simulink model "pll_stability_9bus"  (R2025b)
settings: Solver=ode23t  StartTime=0.0  StopTime=0.6  FixedStep=Ts  RelTol=1e-3  EnableMultiTasking=on
InitFcn:
  | proj_root = fileparts(get_param(bdroot, 'FileName'));
  | run(fullfile(proj_root, 'params.m'))
StopFcn:
  | run(fullfile(fileparts(get_param(bdroot, 'FileName')), 'scripts', 'export_sim_data.m'))
values from neighbouring files (symbols this model uses):
  C1 = 4.247098756978487e-05    (= 4.24709875698e-05)    [GridTiedInverterOptimalIData.m]    (also in params.m)
  den_notch_d = [1.0, -1.9198159829792367, 0.9417686752314415]    [params.m]
  Ki = 7075.557375636462 /4    (= 1768.88934391)    [GridTiedInverterOptimalIData.m]    (also in params.m)
  ki_pll = ki_pll * 0.2    (= 21164)    [params.m]
  Kp = 29.481489065151926 /4    (= 7.37037226629)    [GridTiedInverterOptimalIData.m]    (also in params.m)
  kp_pll = kp_pll * 0.2    (= 92)    [params.m]
  L1 = 0.03042088602562317    (= 0.0304208860256)    [GridTiedInverterOptimalIData.m]    (also in params.m)
  L2 = 0.0002889984172434201    (= 0.000288998417243)    [GridTiedInverterOptimalIData.m]    (also in params.m)
  num_notch_d = [0.9723401207349347, -1.9198159829792367, 0.9694285544965067]    [params.m]
  qsi = 0.707    [GridTiedInverterOptimalIData.m]    (also in params.m)
  Rd1 = 0.5734201923227409    (= 0.573420192323)    [GridTiedInverterOptimalIData.m]    (also in params.m)
  Rd2 = 0.0054474918270660385    (= 0.00544749182707)    [GridTiedInverterOptimalIData.m]    (also in params.m)
  Rd3 = 3.1228169353331086    (= 3.12281693533)    [GridTiedInverterOptimalIData.m]    (also in params.m)
  Ts = 5e-6    (= 5e-06)    [GridTiedInverterOptimalIData.m]    (also in params.m)
  Tsc = 2e-4    (= 0.0002)    [GridTiedInverterOptimalIData.m]    (also in params.m)
  Vcc = 90909.09090909091*1.5    (= 136363.636364)    [GridTiedInverterOptimalIData.m]    (also in params.m)
  wres = 9068.99682117109    (= 9068.99682117)    [GridTiedInverterOptimalIData.m]    (also in params.m)
libraries: nesl_utility x80, ee_lib x71, fl_lib x28, eeGeneralControl x9, eeTransforms x4, eeSmAC1C x3, eeSmPSS1A x3, simulink x3, eeSinusoidalMeasurement x1
(part 2 of 3)

== system pll_stability_9bus/Gen2@Bus2 PV 1.025 pu 163 MW ==
  AVR and Exciter : Subsystem
  Bus Creator : BusCreator  Inputs=3
  Gen2 : ee_lib/Electromechanical/Synchronous/Synchronous Machine Round Rotor  port_option=ee.enum.threePhasePort.composite  SRated=192 MW  VRated=18 kV  FRated=60 Hz  nPolePairs=1  param_option=ee.enum.sm.parameterization.standard  fieldCircuitParameterization_option=ee.enum.sm.fieldparameterization.current  baseEfd=92.95 V  baseIfd=100 A  zero_sequence=ee.enum.park.zerosequence.include  axes_param=ee.enum.rotorangle.qaxis  Ladu=1.6801  Laqu=1.62  L0=0.0399  Ll=0.0399  Ra=0.01  Lfd=0.2162  Rfd=8.558e-4  L1d=0.4343  R1d=0.0325  L1q=0.2635  R1q=0.0326  L2q=0.4627  R2q=0.0131  Xl=0.1  Xd=1.7199  Xq=1.6598  X0=0.1  Xdd=0.23  Xqd=0.378  Xddd=0.1728  Xqdd=0.192  d_option=ee.enum.circuit.open  Td0d=6 s  Tdd=1.3260 s  Td0dd=0.05 s  Tddd=0.0230 s  q_option=ee.enum.circuit.open  Tq0d=0.535 s  Tqd=0.3693 s  Tq0dd=0.04 s  Tqdd=0.0269 s  saturation_option=ee.enum.saturation.exclude  saturation_ifd=[0.0, 0.48, 0.76, 1.38, 1.79]  saturation_Vag=[0.0, 0.8, 1.08, 1.31, 1.4]  initialization_option=ee.enum.sm.initialization.steadystate  source_type=ee.enum.sm.load_flow_source_type.PV  Vmag0=18*1.025 kV  Vang0=0 deg  Pt0=163 MW  Qt0=0 V*A  minimum_pu=0.95  phase_search_range=[-30, 30] deg  gmin=1e-6 S  connection_option=ee.enum.Connection.wye  num_q_dampers=2  rotor_offset=-pi / 2 rad  pu_psid_specify=on  pu_psid_priority=High  pu_psid=0  pu_psid_nominal_specify=off  pu_psid_nominal_value=1  pu_psid_nominal_unit=1  pu_psiq_specify=on  pu_psiq_priority=High  pu_psiq=0  pu_psiq_nominal_specify=off  pu_psiq_nominal_value=1  pu_psiq_nominal_unit=1  pu_psifd_specify=on  pu_psifd_priority=High  pu_psifd=0  pu_psifd_nominal_specify=off  pu_psifd_nominal_value=1  pu_psifd_nominal_unit=1  pu_psi1d_specify=on  pu_psi1d_priority=High  pu_psi1d=0  pu_psi1d_nominal_specify=off  pu_psi1d_nominal_value=1  pu_psi1d_nominal_unit=1  pu_psi1q_specify=on  pu_psi1q_priority=High  pu_psi1q=0  pu_psi1q_nominal_specify=off  pu_psi1q_nominal_value=1  pu_psi1q_nominal_unit=1  pu_psi2q_specify=on  pu_psi2q_priority=High  pu_psi2q=0  pu_psi2q_nominal_specify=off  pu_psi2q_nominal_value=1  pu_psi2q_nominal_unit=1  angular_position_diff_specify=off  angular_position_diff_priority=None  angular_position_diff=0 deg  angular_position_diff_nominal_specify=off  angular_position_diff_nominal_value=1  angular_position_diff_nominal_unit=deg  Tmeas=298.15 K  alpha=3.93e-3 1/K  stator_thermal_mass=100 J/K  rotor_thermal_mass=200 J/K  temperatureA_specify=off  temperatureA_priority=High  temperatureA=25 degC  temperatureA_nominal_specify=off  temperatureA_nominal_value=1  temperatureA_nominal_unit=degC  temperatureB_specify=off  temperatureB_priority=High  temperatureB=25 degC  temperatureB_nominal_specify=off  temperatureB_nominal_value=1  temperatureB_nominal_unit=degC  temperatureC_specify=off  temperatureC_priority=High  temperatureC=25 degC  temperatureC_nominal_specify=off  temperatureC_nominal_value=1  temperatureC_nominal_unit=degC  temperatureR_specify=off  temperatureR_priority=High  temperatureR=25 degC  temperatureR_nominal_specify=off  temperatureR_nominal_value=1  temperatureR_nominal_unit=degC
      settings: InternalSimscapePortConfiguration="{\"Bottom\":[],\"Left\":[{\"id\":\"fd_p\",\"label\":\"fd+\",\"type\":\"foundation.electrical.electrical\"},{\"id\":\"fd_n\",\"label\":\"fd-\",\"type\":\"foundation.electrical.electrical\"},{\"id\":\"R\",\"label\":\"R\",\"type\":\"foundation.mechanical.rotational.rotational\"},{\"id\":\"C\",\"label\":\"C\",\"type\":\"foundation.mechanical.rotational.rotational\"}],\"Right\":[{\"id\":\"pu_output\",\"label\":\"pu\",\"type\":\"output\"},{\"id\":\"N\",\"label\":\"~\",\"type\":\"foundation.electrical.three_phase\"},{\"id\":\"n\",\"label\":\"n\",\"type\":\"foundation.electrical.electrical\"}],\"Top\":[]}"
  Gnd : fl_lib/Electrical/Electrical Elements/Electrical Reference
  Governor and Prime Mover : Subsystem
  PS-Simulink Converter1 : nesl_utility/PS-Simulink Converter  PhysicalDomain=network_engine_domain  SubClassName=ps_output  LeftPortType=input  RightPortType=output  PseudoPeriodic=off  Frequencies=[]  VectorFormat=1-D array  Unit=1  AffineConversion=off
  PS-Simulink Converter11 : nesl_utility/PS-Simulink Converter  PhysicalDomain=network_engine_domain  SubClassName=ps_output  LeftPortType=input  RightPortType=output  PseudoPeriodic=off  Frequencies=[]  VectorFormat=1-D array  Unit=1  AffineConversion=off
  PS-Simulink Converter12 : nesl_utility/PS-Simulink Converter  PhysicalDomain=network_engine_domain  SubClassName=ps_output  LeftPortType=input  RightPortType=output  PseudoPeriodic=off  Frequencies=[]  VectorFormat=1-D array  Unit=1  AffineConversion=off
  Rotor electrical angle : ee_lib/Electromechanical/Synchronous/Synchronous Machine Measurement  output_idx=19
      settings: InternalSimscapePortConfiguration="{\"Bottom\":[],\"Left\":[{\"id\":\"pu_input\",\"label\":\"pu\",\"type\":\"input\"}],\"Right\":[{\"id\":\"pu_output\",\"label\":\"o\",\"type\":\"output\"}],\"Top\":[]}"
  Rotor velocity : ee_lib/Electromechanical/Synchronous/Synchronous Machine Measurement  output_idx=4
      settings: InternalSimscapePortConfiguration="{\"Bottom\":[],\"Left\":[{\"id\":\"pu_input\",\"label\":\"pu\",\"type\":\"input\"}],\"Right\":[{\"id\":\"pu_output\",\"label\":\"o\",\"type\":\"output\"}],\"Top\":[]}"
  Terminal voltage : ee_lib/Electromechanical/Synchronous/Synchronous Machine Measurement  output_idx=14
      settings: InternalSimscapePortConfiguration="{\"Bottom\":[],\"Left\":[{\"id\":\"pu_input\",\"label\":\"pu\",\"type\":\"input\"}],\"Right\":[{\"id\":\"pu_output\",\"label\":\"o\",\"type\":\"output\"}],\"Top\":[]}"
  ConnGen : PMIOPort  Side=Right
  mGen : Outport
  wires:
  PS-Simulink Converter11/1 -> Bus Creator/1  "w"
  Bus Creator/1 -> mGen/1
  PS-Simulink Converter12/1 -> Bus Creator/2  "Vt"
  PS-Simulink Converter1/1 -> Bus Creator/3  "theta"
  connections:
  AVR and Exciter/RConn1 -- Gen2/LConn1
  AVR and Exciter/RConn2 -- Gen2/LConn2
  Gen2/LConn3 -- Governor and Prime Mover/RConn1
  Gen2/LConn4 -- Governor and Prime Mover/RConn2
  Gen2/RConn2 -- ConnGen/RConn1
  Gen2/RConn3 -- Gnd/LConn1
  Gen2/RConn1 -- AVR and Exciter/LConn1 -- Governor and Prime Mover/LConn1 -- Rotor electrical angle/LConn1 -- Rotor velocity/LConn1 -- Terminal voltage/LConn1
  PS-Simulink Converter11/LConn1 -- Rotor velocity/RConn1
  PS-Simulink Converter12/LConn1 -- Terminal voltage/RConn1
  Rotor electrical angle/RConn1 -- PS-Simulink Converter1/LConn1

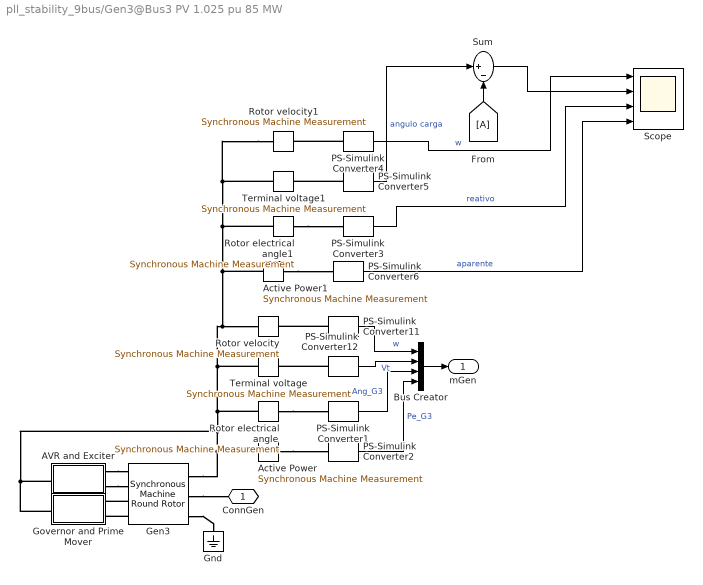
== system pll_stability_9bus/Gen3@Bus3 PV 1.025 pu 85 MW ==
  AVR and Exciter : Subsystem
  Active Power : ee_lib/Electromechanical/Synchronous/Synchronous Machine Measurement  output_idx=12
      settings: InternalSimscapePortConfiguration="{\"Bottom\":[],\"Left\":[{\"id\":\"pu_input\",\"label\":\"pu\",\"type\":\"input\"}],\"Right\":[{\"id\":\"pu_output\",\"label\":\"o\",\"type\":\"output\"}],\"Top\":[]}"
  Active Power1 : ee_lib/Electromechanical/Synchronous/Synchronous Machine Measurement  output_idx=11
      settings: InternalSimscapePortConfiguration="{\"Bottom\":[],\"Left\":[{\"id\":\"pu_input\",\"label\":\"pu\",\"type\":\"input\"}],\"Right\":[{\"id\":\"pu_output\",\"label\":\"o\",\"type\":\"output\"}],\"Top\":[]}"
  Bus Creator : BusCreator  Inputs=4
  From : From
  Gen3 : ee_lib/Electromechanical/Synchronous/Synchronous Machine Round Rotor  port_option=ee.enum.threePhasePort.composite  SRated=128 MW  VRated=13.8 kV  FRated=60 Hz  nPolePairs=1  param_option=ee.enum.sm.parameterization.standard  fieldCircuitParameterization_option=ee.enum.sm.fieldparameterization.current  baseEfd=92.95 V  baseIfd=100 A  zero_sequence=ee.enum.park.zerosequence.include  axes_param=ee.enum.rotorangle.qaxis  Ladu=1.5958  Laqu=1.5257  L0=0.0842  Ll=0.0842  Ra=0.01  Lfd=0.1715  Rfd=8.4749e-4  L1d=0.061  R1d=0.0108  L1q=0.1726  R1q=0.0222  L2q=0.3535  R2q=0.0144  Xl=0.095  Xd=1.68  Xq=1.61  X0=0.095  Xdd=0.2321  Xqd=0.32  Xddd=0.128  Xqdd=0.192  d_option=ee.enum.circuit.open  Td0d=5.89 s  Tdd=1.3260 s  Td0dd=0.05 s  Tddd=0.0230 s  q_option=ee.enum.circuit.open  Tq0d=0.6 s  Tqd=0.3693 s  Tq0dd=0.04 s  Tqdd=0.0269 s  saturation_option=ee.enum.saturation.exclude  saturation_ifd=[0.0, 0.48, 0.76, 1.38, 1.79]  saturation_Vag=[0.0, 0.8, 1.08, 1.31, 1.4]  initialization_option=ee.enum.sm.initialization.steadystate  source_type=ee.enum.sm.load_flow_source_type.PV  Vmag0=13.8*1.025 kV  Vang0=0 deg  Pt0=85 MW  Qt0=0 V*A  minimum_pu=0.95  phase_search_range=[-30, 30] deg  gmin=1e-6 S  connection_option=ee.enum.Connection.wye  num_q_dampers=2  rotor_offset=-pi / 2 rad  pu_psid_specify=on  pu_psid_priority=High  pu_psid=0  pu_psid_nominal_specify=off  pu_psid_nominal_value=1  pu_psid_nominal_unit=1  pu_psiq_specify=on  pu_psiq_priority=High  pu_psiq=0  pu_psiq_nominal_specify=off  pu_psiq_nominal_value=1  pu_psiq_nominal_unit=1  pu_psifd_specify=on  pu_psifd_priority=High  pu_psifd=0  pu_psifd_nominal_specify=off  pu_psifd_nominal_value=1  pu_psifd_nominal_unit=1  pu_psi1d_specify=on  pu_psi1d_priority=High  pu_psi1d=0  pu_psi1d_nominal_specify=off  pu_psi1d_nominal_value=1  pu_psi1d_nominal_unit=1  pu_psi1q_specify=on  pu_psi1q_priority=High  pu_psi1q=0  pu_psi1q_nominal_specify=off  pu_psi1q_nominal_value=1  pu_psi1q_nominal_unit=1  pu_psi2q_specify=on  pu_psi2q_priority=High  pu_psi2q=0  pu_psi2q_nominal_specify=off  pu_psi2q_nominal_value=1  pu_psi2q_nominal_unit=1  angular_position_diff_specify=off  angular_position_diff_priority=High  angular_position_diff=0 deg  angular_position_diff_nominal_specify=off  angular_position_diff_nominal_value=1  angular_position_diff_nominal_unit=deg  Tmeas=298.15 K  alpha=3.93e-3 1/K  stator_thermal_mass=100 J/K  rotor_thermal_mass=200 J/K  temperatureA_specify=off  temperatureA_priority=High  temperatureA=25 degC  temperatureA_nominal_specify=off  temperatureA_nominal_value=1  temperatureA_nominal_unit=degC  temperatureB_specify=off  temperatureB_priority=High  temperatureB=25 degC  temperatureB_nominal_specify=off  temperatureB_nominal_value=1  temperatureB_nominal_unit=degC  temperatureC_specify=off  temperatureC_priority=High  temperatureC=25 degC  temperatureC_nominal_specify=off  temperatureC_nominal_value=1  temperatureC_nominal_unit=degC  temperatureR_specify=off  temperatureR_priority=High  temperatureR=25 degC  temperatureR_nominal_specify=off  temperatureR_nominal_value=1  temperatureR_nominal_unit=degC
      settings: InternalSimscapePortConfiguration="{\"Bottom\":[],\"Left\":[{\"id\":\"fd_p\",\"label\":\"fd+\",\"type\":\"foundation.electrical.electrical\"},{\"id\":\"fd_n\",\"label\":\"fd-\",\"type\":\"foundation.electrical.electrical\"},{\"id\":\"R\",\"label\":\"R\",\"type\":\"foundation.mechanical.rotational.rotational\"},{\"id\":\"C\",\"label\":\"C\",\"type\":\"foundation.mechanical.rotational.rotational\"}],\"Right\":[{\"id\":\"pu_output\",\"label\":\"pu\",\"type\":\"output\"},{\"id\":\"N\",\"label\":\"~\",\"type\":\"foundation.electrical.three_phase\"},{\"id\":\"n\",\"label\":\"n\",\"type\":\"foundation.electrical.electrical\"}],\"Top\":[]}"
  Gnd : fl_lib/Electrical/Electrical Elements/Electrical Reference
  Governor and Prime Mover : Subsystem
  PS-Simulink Converter{1..6,11..12} (8 alike) : nesl_utility/PS-Simulink Converter  PhysicalDomain=network_engine_domain  SubClassName=ps_output  LeftPortType=input  RightPortType=output  PseudoPeriodic=off  Frequencies=[]  VectorFormat=1-D array  Unit=1  AffineConversion=off
  Rotor electrical angle : ee_lib/Electromechanical/Synchronous/Synchronous Machine Measurement  output_idx=19
      settings: InternalSimscapePortConfiguration="{\"Bottom\":[],\"Left\":[{\"id\":\"pu_input\",\"label\":\"pu\",\"type\":\"input\"}],\"Right\":[{\"id\":\"pu_output\",\"label\":\"o\",\"type\":\"output\"}],\"Top\":[]}"
  Rotor electrical angle1 : ee_lib/Electromechanical/Synchronous/Synchronous Machine Measurement  output_idx=13
      settings: InternalSimscapePortConfiguration="{\"Bottom\":[],\"Left\":[{\"id\":\"pu_input\",\"label\":\"pu\",\"type\":\"input\"}],\"Right\":[{\"id\":\"pu_output\",\"label\":\"o\",\"type\":\"output\"}],\"Top\":[]}"
  Rotor velocity : ee_lib/Electromechanical/Synchronous/Synchronous Machine Measurement  output_idx=4
      settings: InternalSimscapePortConfiguration="{\"Bottom\":[],\"Left\":[{\"id\":\"pu_input\",\"label\":\"pu\",\"type\":\"input\"}],\"Right\":[{\"id\":\"pu_output\",\"label\":\"o\",\"type\":\"output\"}],\"Top\":[]}"
  Rotor velocity1 : ee_lib/Electromechanical/Synchronous/Synchronous Machine Measurement  output_idx=4
      settings: InternalSimscapePortConfiguration="{\"Bottom\":[],\"Left\":[{\"id\":\"pu_input\",\"label\":\"pu\",\"type\":\"input\"}],\"Right\":[{\"id\":\"pu_output\",\"label\":\"o\",\"type\":\"output\"}],\"Top\":[]}"
  Scope : Scope  NumInputPorts=4
      settings: ActiveDisplayYMinimum=0.992134056706686  ActiveDisplayYMaximum=1.0008746376390321  DataLoggingVariableName=ScopeData28
  Sum : Sum  Inputs=|+-
  Terminal voltage : ee_lib/Electromechanical/Synchronous/Synchronous Machine Measurement  output_idx=14
      settings: InternalSimscapePortConfiguration="{\"Bottom\":[],\"Left\":[{\"id\":\"pu_input\",\"label\":\"pu\",\"type\":\"input\"}],\"Right\":[{\"id\":\"pu_output\",\"label\":\"o\",\"type\":\"output\"}],\"Top\":[]}"
  Terminal voltage1 : ee_lib/Electromechanical/Synchronous/Synchronous Machine Measurement  output_idx=18
      settings: InternalSimscapePortConfiguration="{\"Bottom\":[],\"Left\":[{\"id\":\"pu_input\",\"label\":\"pu\",\"type\":\"input\"}],\"Right\":[{\"id\":\"pu_output\",\"label\":\"o\",\"type\":\"output\"}],\"Top\":[]}"
  ConnGen : PMIOPort  Side=Right
  mGen : Outport
  wires:
  PS-Simulink Converter1/1 -> Bus Creator/3  "Ang_G3"
  PS-Simulink Converter12/1 -> Bus Creator/2  "Vt"
  Bus Creator/1 -> mGen/1
  PS-Simulink Converter11/1 -> Bus Creator/1  "w"
  PS-Simulink Converter2/1 -> Bus Creator/4  "Pe_G3"
  PS-Simulink Converter5/1 -> Sum/1  "angulo carga"
  PS-Simulink Converter4/1 -> Scope/1  "w"
  PS-Simulink Converter3/1 -> Scope/3  "reativo"
  PS-Simulink Converter6/1 -> Scope/4  "aparente"
  From/1 -> Sum/2
  Sum/1 -> Scope/2
  connections:
  Rotor electrical angle/RConn1 -- PS-Simulink Converter1/LConn1
  PS-Simulink Converter12/LConn1 -- Terminal voltage/RConn1
  PS-Simulink Converter11/LConn1 -- Rotor velocity/RConn1
  Rotor velocity1/LConn1 -- Terminal voltage1/LConn1 -- Rotor electrical angle1/LConn1 -- Rotor velocity/LConn1 -- Terminal voltage/LConn1 -- Gen3/RConn1 -- Active Power/LConn1 -- AVR and Exciter/LConn1 -- Governor and Prime Mover/LConn1 -- Rotor electrical angle/LConn1 -- Active Power1/LConn1
  Gen3/RConn3 -- Gnd/LConn1
  Gen3/RConn2 -- ConnGen/RConn1
  Gen3/LConn4 -- Governor and Prime Mover/RConn2
  Gen3/LConn3 -- Governor and Prime Mover/RConn1
  AVR and Exciter/RConn2 -- Gen3/LConn2
  AVR and Exciter/RConn1 -- Gen3/LConn1
  Active Power/RConn1 -- PS-Simulink Converter2/LConn1
  Active Power1/RConn1 -- PS-Simulink Converter6/LConn1
  PS-Simulink Converter4/LConn1 -- Rotor velocity1/RConn1
  PS-Simulink Converter5/LConn1 -- Terminal voltage1/RConn1
  Rotor electrical angle1/RConn1 -- PS-Simulink Converter3/LConn1

== system pll_stability_9bus/Scope ==
  BusElementIn : Inport  PortName=mGen1  Element=w
  BusElementIn1 : Inport  PortName=mGen1  Element=Vt
  BusElementIn3 : Inport  Port=2  PortName=mGen3  Element=Vt
  BusElementIn5 : Inport  Port=2  PortName=mGen3  Element=w
  Mux : Mux  Inputs=2
  Mux1 : Mux  Inputs=2
  Scope : Scope  NumInputPorts=2
      settings: ActiveDisplayYMinimum=0.30512027523637242  ActiveDisplayYMaximum=1.3392045145647005
  wires:
  BusElementIn/1 -> Mux/1
  BusElementIn1/1 -> Mux1/1
  BusElementIn3/1 -> Mux1/2
  Mux1/1 -> Scope/1  "Terminal voltages [p.u.]"
  Mux/1 -> Scope/2  "Rotor speeds [p.u.]"
  BusElementIn5/1 -> Mux/2

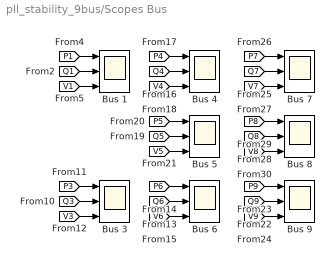
== system pll_stability_9bus/Scopes Bus ==
  Bus {1,3..9} (8 alike) : Scope  NumInputPorts=3
      Bus 1 settings: ActiveDisplayYMinimum=-49.114456824665893  ActiveDisplayYMaximum=442.03011142199318  DataLoggingVariableName=ScopeData11
      Bus 3 settings: ActiveDisplayYMinimum=-59.99075912656123  ActiveDisplayYMaximum=266.60428494941306  DataLoggingVariableName=ScopeData10
      Bus 4 settings: ActiveDisplayYMinimum=-38.55667965898116  ActiveDisplayYMaximum=347.01011693083052  DataLoggingVariableName=ScopeData14
      Bus 5 settings: ActiveDisplayYMinimum=-192.77982685772625  ActiveDisplayYMaximum=116.10526480167731  DataLoggingVariableName=ScopeData12
      Bus 6 settings: ActiveDisplayYMinimum=-45.726697361068808  ActiveDisplayYMaximum=76.089380993056864  DataLoggingVariableName=ScopeData13
      Bus 7 settings: ActiveDisplayYMinimum=-344.11330563303079  ActiveDisplayYMaximum=223.61219150109264  DataLoggingVariableName=ScopeData17
      Bus 8 settings: ActiveDisplayYMinimum=-150.38081880811259  ActiveDisplayYMaximum=115.04879751678179  DataLoggingVariableName=ScopeData15
      Bus 9 settings: ActiveDisplayYMinimum=-29.497454320573244  ActiveDisplayYMaximum=265.47708888515928  DataLoggingVariableName=ScopeData16
  wires:
  [V4] -> Bus 4/3
  [Q9] -> Bus 9/2
  [V6] -> Bus 6/3
  [V9] -> Bus 9/3
  [P5] -> Bus 5/1
  [Q1] -> Bus 1/2
  [Q8] -> Bus 8/2
  [P6] -> Bus 6/1
  [P4] -> Bus 4/1
  [V5] -> Bus 5/3
  [P9] -> Bus 9/1
  [V1] -> Bus 1/3
  [Q5] -> Bus 5/2
  [P7] -> Bus 7/1
  [Q6] -> Bus 6/2
  [Q4] -> Bus 4/2
  [P8] -> Bus 8/1
  [P1] -> Bus 1/1
  [V8] -> Bus 8/3
  [V7] -> Bus 7/3
  [Q7] -> Bus 7/2
  [Q3] -> Bus 3/2
  [P3] -> Bus 3/1
  [V3] -> Bus 3/3

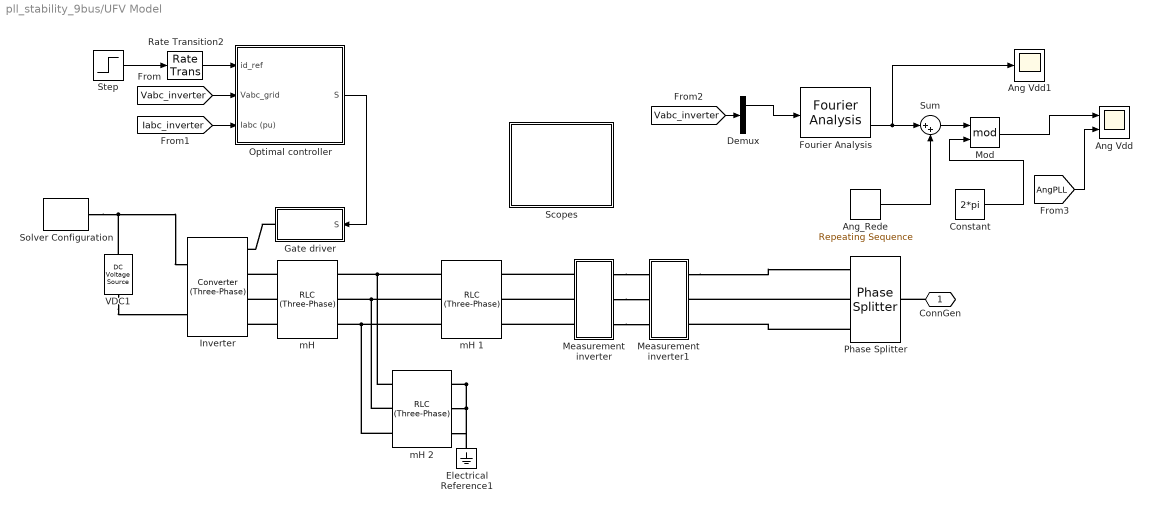
== system pll_stability_9bus/UFV Model ==
  " mH " : ee_lib/Passive/RLC Assemblies/RLC (Three-Phase)  port_option=ee.enum.threePhasePort.expanded  component_structure=ee.enum.rlc.structure.SeriesRL  R=Rd1 Ohm  L=L1 H  C=1 F  R_parasitic=1e-6 Ohm  G_parasitic=1e-6 1/Ohm  IL_specify=on  IL_priority=High  IL=[0, 0, 0] A  IL_nominal_specify=off  IL_nominal_value=1  IL_nominal_unit=A  VC_specify=on  VC_priority=High  VC=[0, 0, 0] V  VC_nominal_specify=off  VC_nominal_value=1  VC_nominal_unit=V
      settings: InternalSimscapePortConfiguration="{\"Bottom\":[],\"Left\":[{\"id\":\"a1\",\"label\":\"a1\",\"type\":\"foundation.electrical.electrical\"},{\"id\":\"b1\",\"label\":\"b1\",\"type\":\"foundation.electrical.electrical\"},{\"id\":\"c1\",\"label\":\"c1\",\"type\":\"foundation.electrical.electrical\"}],\"Right\":[{\"id\":\"a2\",\"label\":\"a2\",\"type\":\"foundation.electrical.electrical\"},{\"id\":\"b2\",\"label\":\"b2\",\"type\":\"foundation.electrical.electrical\"},{\"id\":\"c2\",\"label\":\"c2\",\"type\":\"foundation.electrical.electrical\"}],\"Top\":[]}"
  " mH 1" : ee_lib/Passive/RLC Assemblies/RLC (Three-Phase)  port_option=ee.enum.threePhasePort.expanded  component_structure=ee.enum.rlc.structure.SeriesRL  R=Rd2 Ohm  L=L2 H  C=1 F  R_parasitic=1e-6 Ohm  G_parasitic=1e-6 1/Ohm  IL_specify=on  IL_priority=High  IL=[0, 0, 0] A  IL_nominal_specify=off  IL_nominal_value=1  IL_nominal_unit=A  VC_specify=on  VC_priority=High  VC=[0, 0, 0] V  VC_nominal_specify=off  VC_nominal_value=1  VC_nominal_unit=V
      settings: InternalSimscapePortConfiguration="{\"Bottom\":[],\"Left\":[{\"id\":\"a1\",\"label\":\"a1\",\"type\":\"foundation.electrical.electrical\"},{\"id\":\"b1\",\"label\":\"b1\",\"type\":\"foundation.electrical.electrical\"},{\"id\":\"c1\",\"label\":\"c1\",\"type\":\"foundation.electrical.electrical\"}],\"Right\":[{\"id\":\"a2\",\"label\":\"a2\",\"type\":\"foundation.electrical.electrical\"},{\"id\":\"b2\",\"label\":\"b2\",\"type\":\"foundation.electrical.electrical\"},{\"id\":\"c2\",\"label\":\"c2\",\"type\":\"foundation.electrical.electrical\"}],\"Top\":[]}"
  " mH 2" : ee_lib/Passive/RLC Assemblies/RLC (Three-Phase)  port_option=ee.enum.threePhasePort.expanded  component_structure=ee.enum.rlc.structure.ParallelRC  R=Rd3 Ohm  L=0.002 H  C=C1 F  R_parasitic=1e-6 Ohm  G_parasitic=1e-6 1/Ohm  IL_specify=on  IL_priority=High  IL=[0, 0, 0] A  IL_nominal_specify=off  IL_nominal_value=1  IL_nominal_unit=A  VC_specify=on  VC_priority=High  VC=[0, 0, 0] V  VC_nominal_specify=off  VC_nominal_value=1  VC_nominal_unit=V
      settings: InternalSimscapePortConfiguration="{\"Bottom\":[],\"Left\":[{\"id\":\"a1\",\"label\":\"a1\",\"type\":\"foundation.electrical.electrical\"},{\"id\":\"b1\",\"label\":\"b1\",\"type\":\"foundation.electrical.electrical\"},{\"id\":\"c1\",\"label\":\"c1\",\"type\":\"foundation.electrical.electrical\"}],\"Right\":[{\"id\":\"a2\",\"label\":\"a2\",\"type\":\"foundation.electrical.electrical\"},{\"id\":\"b2\",\"label\":\"b2\",\"type\":\"foundation.electrical.electrical\"},{\"id\":\"c2\",\"label\":\"c2\",\"type\":\"foundation.electrical.electrical\"}],\"Top\":[]}"
  Ang Vdd : Scope  NumInputPorts=2
      settings: ActiveDisplayYMinimum=-0.78537822507117583  ActiveDisplayYMaximum=7.068404025640584  DataLoggingVariableName=ScopeData8
  Ang Vdd1 : Scope
      settings: ActiveDisplayYMinimum=-3.9268785604995653  ActiveDisplayYMaximum=3.9266971999008624  DataLoggingVariableName=ScopeData25
  Ang_Rede : simulink/Sources/Repeating Sequence  rep_seq_t=[0 1/60]  rep_seq_y=[0 2*pi]
  Constant : Constant  Value=2*pi
  Demux : Demux  Outputs=3
  Electrical Reference1 : fl_lib/Electrical/Electrical Elements/Electrical Reference
  Fourier Analysis : eeGeneralControl/Fourier Analysis  f=60  n=[1]  M0=1  Ph0=0  BufferSize=8192  Ts=-1
      settings: LibrarySourceBlock=ee_sl_lib/General Control/Fourier Analysis
  Gate driver : Subsystem
  Inverter : ee_lib/Semiconductors & Converters/Converters/Converter (Three-Phase)  port_option=ee.enum.threePhasePort.expanded  fidelity_option=ee.enum.converters.fidelity.detailed  device_type=ee.enum.converters.switchingdevice.ideal  showThermalPort=false  K=0  Vth=0.5 V  Vgt=1e-3 V  Vgt_off=-1 V  Ih=1 A  Vf=0.8 V  Ron=1e-3 Ohm  Rds=0.001 Ohm  Goff=2e-4 1/Ohm  Eon_scalar=22.86e-3 J  Eoff_scalar=17.14e-3 J  Eoff_natural_commutation=10e-3 J  Voff=300 V  Iout_scalar=600 A  onCurrentMeasDelay=0 s  useCurrentFromPreviousCycle=false  useVoltageFromPreviousCycle=false  diode_param=ee.enum.converters.protectiondiode.nodynamics  diode_Vf=0.8 V  diode_Ron=0.001 Ohm  diode_Goff=1e-5 1/Ohm  diode_C=50 nF  diode_iRM=-235 A  diode_iF=300 A  diode_idot=-50 A/us  diode_trr_param=ee.enum.converters.diodetrr.trr_factor  diode_trr_factor=3  diode_trr=15 us  diode_Qrr=1.5e+3 s*uA  diode_rec_loss_model=ee.enum.diode.reverseRecoveryModel.fixed  diode_ErecVal=0 J  diode_scaleWithIandV=false  diode_ErecMat=zeros(2, 3) J  diode_TjrecVec=[298.15, 398.15] K  diode_IfrecVec=[.1, 1, 10] A  diode_IrecVal=10 A  diode_VrecVal=10 V  diode_tFilter=1 / 1000 / 100 s  thermal_network_parameterization=ee.enum.thermalNetworkTopology.external  Rth=[.08, .5] K/W  Rth_Cauer=[.08, .1, .5] K/W  Rth_Foster=[.08, .14, .22, .16] K/W  thermal_mass_parameterization=ee.enum.thermalNetwork.timeconstant  thermal_mass=[.01, .5] J/K  thermal_mass_Cauer=[.01, .1, .5] J/K  thermal_mass_Foster=[.001, .005, .05, .5] J/K  thermal_time_constant=[.001, .2] s  thermal_time_constant_Cauer=[.001, .1, .2] s  thermal_time_constant_Foster=[7e-05, .0007, .01, .08] s  thermal_mass_initial_temperatures=[25, 25] degC  thermal_mass_initial_temperatures_Cauer=[25, 25, 25] degC  junction_thermal_mass=0.01 J/K  Tvec_initial_Foster=[25, 25, 25, 25] degC  snubber_type=ee.enum.converters.snubber.exclude  Cs=1e-7 F  Rs=0.1 Ohm  Vce_loss=[0, 150, 300] V
      settings: InternalSimscapePortConfiguration="{\"Bottom\":[],\"Left\":[{\"id\":\"G\",\"label\":\"G\",\"type\":\"foundation.electrical.twelve_phase\"},{\"id\":\"a\",\"label\":\"a\",\"type\":\"foundation.electrical.electrical\"},{\"id\":\"b\",\"label\":\"b\",\"type\":\"foundation.electrical.electrical\"},{\"id\":\"c\",\"label\":\"c\",\"type\":\"foundation.electrical.electrical\"}],\"Right\":[{\"id\":\"p\",\"label\":\"+\",\"type\":\"foundation.electrical.electrical\"},{\"id\":\"n\",\"label\":\"-\",\"type\":\"foundation.electrical.electrical\"}],\"Top\":[]}"
  Measurement inverter : Subsystem
  Measurement inverter1 : Subsystem
  Mod : Math  Operator=mod
  Optimal controller : Subsystem
  Phase Splitter : ee_lib/Connectors & References/Phase Splitter
  Rate Transition2 : RateTransition  OutPortSampleTime=Tsc
  Scopes : Subsystem
  Solver Configuration : nesl_utility/Solver Configuration  PhysicalDomain=network_engine_domain  SubClassName=solver  LeftPortType=input  RightPortType=generic  Tones=[]  Harmonics=[]  SimulateNoise=off  Profile=off  UseLocalSampling=off  EnableSwitchedLinearOptims=on  FrequencyDomain=off  UseCCode=off  RelTol=0.001  AbsTol=1e-06  MinStep=1e-09  ToWorkspace=off  RevertToSquareIcSolve=off  NumHomotopyIterations=100  PhasorMode=off  PhasorModeNumHarmonics=1  ConsistencySolver=NEWTON_FTOL  IndexReductionMethod=DerivativeReplacement  DoDC=off  ResidualTolerance=1e-09  ConsistencyTolSource=GLOBAL  ConsistencyAbsTol=0.001  ConsistencyRelTol=0.001  ConsistencyTolFactor=0.001  UseLocalSolver=on  LocalSolverChoice=NE_BACKWARD_EULER_ADVANCER  ResolveIndetEquations=on  FunctionEvalNumThread=1  LocalSolverSampleTime=Ts  DoFixedCost=off  MaxNonlinIter=3  MaxModeIter=2  ComputeImpulses=off  ImpulseIterations=1  LinearAlgebra=auto  LinearAlgebraNumThread=0  EquationFormulation=NE_TIME_EF  DelaysMemoryBudget=1024  AutomaticFiltering=on  FilteringTimeConstant=0.001  PartitionStorageMethod=AS_NEEDED  PartitionMemoryBudget=1024  PartitionMethod=FAST  MultibodyUseLocalSolver=off  MultibodyLocalSolverChoice=ODE1  MultibodyLocalSolverSampleTime=0.001
  Step : Step  Time=0.01  SampleTime=0
  Sum : Sum  Inputs=|++
  VDC1 : fl_lib/Electrical/Electrical Sources/DC Voltage Source  v0=Vcc*1.7 V
  ConnGen : PMIOPort  Side=Right
  wires:
  [Iabc_inverter] -> Optimal controller/3(Iabc (pu))
  [Vabc_inverter] -> Optimal controller/2(Vabc_grid)
  Rate Transition2/1 -> Optimal controller/1(id_ref)
  Step/1 -> Rate Transition2/1
  Optimal controller/1(S) -> Gate driver/1(S)
  [Vabc_inverter] -> Demux/1
  Demux/1 -> Fourier Analysis/1
  Fourier Analysis/2 -> Ang Vdd1/1, Sum/1
  Ang_Rede/1 -> Sum/2
  Sum/1 -> Mod/1
  Mod/1 -> Ang Vdd/1
  Constant/1 -> Mod/2
  [AngPLL] -> Ang Vdd/2
  connections:
  " mH 2"/LConn3 -- " mH "/RConn3 -- " mH 1"/LConn3
  " mH 2"/RConn1 -- " mH 2"/RConn2 -- Electrical Reference1/LConn1 -- " mH 2"/RConn3
  " mH 2"/LConn2 -- " mH "/RConn2 -- " mH 1"/LConn2
  Measurement inverter/LConn3 -- " mH 1"/RConn3
  " mH "/LConn2 -- Inverter/LConn3
  Solver Configuration/RConn1 -- Inverter/RConn1 -- VDC1/LConn1
  " mH 2"/LConn1 -- " mH "/RConn1 -- " mH 1"/LConn1
  Measurement inverter/RConn1 -- Measurement inverter1/LConn1
  Measurement inverter/RConn3 -- Measurement inverter1/LConn3
  " mH "/LConn1 -- Inverter/LConn2
  Measurement inverter/LConn1 -- " mH 1"/RConn1
  Gate driver/RConn1 -- Inverter/LConn1
  Phase Splitter/RConn3 -- Measurement inverter1/RConn3
  VDC1/RConn1 -- Inverter/RConn2
  " mH "/LConn3 -- Inverter/LConn4
  Measurement inverter1/RConn1 -- Phase Splitter/RConn1
  Phase Splitter/RConn2 -- Measurement inverter1/RConn2
  Measurement inverter/RConn2 -- Measurement inverter1/LConn2
  Measurement inverter/LConn2 -- " mH 1"/RConn2
  ConnGen/RConn1 -- Phase Splitter/LConn1

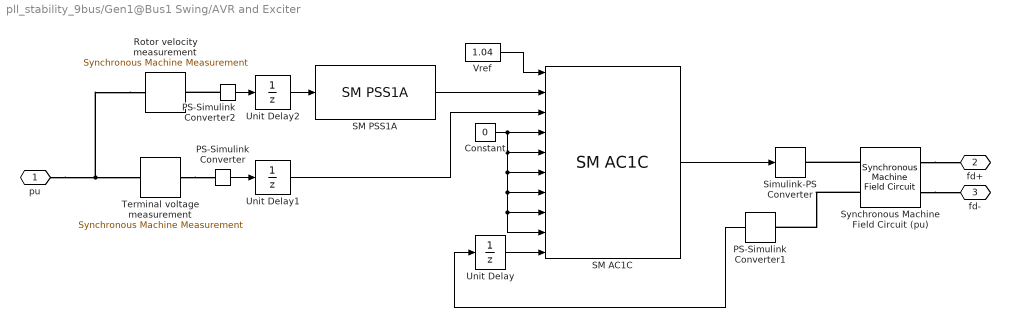
== system pll_stability_9bus/Gen1@Bus1 Swing/AVR and Exciter ==
  Constant : Constant  Value=0
  PS-Simulink Converter : nesl_utility/PS-Simulink Converter  PhysicalDomain=network_engine_domain  SubClassName=ps_output  LeftPortType=input  RightPortType=output  PseudoPeriodic=off  Frequencies=[]  VectorFormat=1-D array  Unit=1  AffineConversion=off
  PS-Simulink Converter1 : nesl_utility/PS-Simulink Converter  PhysicalDomain=network_engine_domain  SubClassName=ps_output  LeftPortType=input  RightPortType=output  PseudoPeriodic=off  Frequencies=[]  VectorFormat=1-D array  Unit=1  AffineConversion=off
  PS-Simulink Converter2 : nesl_utility/PS-Simulink Converter  PhysicalDomain=network_engine_domain  SubClassName=ps_output  LeftPortType=input  RightPortType=output  PseudoPeriodic=off  Frequencies=[]  VectorFormat=1-D array  Unit=1  AffineConversion=off
  Rotor velocity measurement : ee_lib/Electromechanical/Synchronous/Synchronous Machine Measurement  output_idx=4
      settings: InternalSimscapePortConfiguration="{\"Bottom\":[],\"Left\":[{\"id\":\"pu_input\",\"label\":\"pu\",\"type\":\"input\"}],\"Right\":[{\"id\":\"pu_output\",\"label\":\"o\",\"type\":\"output\"}],\"Top\":[]}"
  SM AC1C : eeSmAC1C/SM AC1C  E_FD0=1.08614  Ts=Ts  R_C=0  X_C=0  T_R=0  K_A=400  T_A=0.02  T_B=0  T_C=0  K_F=0.03  T_F=1  V_Amax=14.5  V_Amin=-14.5  E_FEmax=6.03  E_FEmin=-5.43  oelInputLocation=Unused  uelInputLocation=Unused  sclInputLocation=Unused  K_E=1  T_E=0.8  K_C=0.2  K_D=0.38  E_1=4.18  S_E_E1=0.1  E_2=3.14  S_E_E2=0.03  V_FEmax=99  V_Emin=0
  SM PSS1A : eeSmPSS1A/SM PSS1A  K_S=3.15  A_1=0  A_2=0  T_1=0  T_2=0  T_3=0.32  T_4=0.016  T_5=1  T_6=0.0106  V_STmax=0.09  V_STmin=-0.09  Ts=Ts
  Simulink-PS Converter : nesl_utility/Simulink-PS Converter  PhysicalDomain=network_engine_domain  SubClassName=ps_input  LeftPortType=input  RightPortType=output  PseudoPeriodic=off  Frequencies=[]  NoiseDistribution=none  NoiseParameters=[]  Unit=1  AffineConversion=off  FilteringAndDerivatives=provide  SimscapeFilterOrder=1  InputFilterTimeConstant=0.001  UdotUserProvided=0
  Synchronous Machine Field Circuit (pu) : ee_lib/Electromechanical/Synchronous/Synchronous Machine Field Circuit  unit_option=ee.enum.unit.pu  SRated=247.5 MW  FRated=60 Hz  fieldCircuitParameterization_option=ee.enum.sm.fieldparameterization.current  baseEfd=92.95 V  baseIfd=100 A  parameterization_option=ee.enum.sm.parameterization.standard  Ladu=0.2725  Rfd=1.0656e-4  Xl=0.0832  Xd=0.3614  Xdd=0.1505  Xddd=0.0990  d_option=ee.enum.circuit.open  Td0d=8.96 s  Tdd=1.3260 s  Td0dd=0.05 s  Tddd=0.0230 s
      settings: InternalSimscapePortConfiguration="{\"Bottom\":[],\"Left\":[{\"id\":\"Efd_pu\",\"label\":\"Efd_pu\",\"type\":\"input\"},{\"id\":\"Ifd_pu\",\"label\":\"Ifd_pu\",\"type\":\"output\"}],\"Right\":[{\"id\":\"fd_p\",\"label\":\"fd+\",\"type\":\"foundation.electrical.electrical\"},{\"id\":\"fd_n\",\"label\":\"fd-\",\"type\":\"foundation.electrical.electrical\"}],\"Top\":[]}"
  Terminal voltage measurement : ee_lib/Electromechanical/Synchronous/Synchronous Machine Measurement  output_idx=14
      settings: InternalSimscapePortConfiguration="{\"Bottom\":[],\"Left\":[{\"id\":\"pu_input\",\"label\":\"pu\",\"type\":\"input\"}],\"Right\":[{\"id\":\"pu_output\",\"label\":\"o\",\"type\":\"output\"}],\"Top\":[]}"
  Unit Delay : UnitDelay  InitialCondition=1.08614  SampleTime=Ts  HasFrameUpgradeWarning=on
  Unit Delay1 : UnitDelay  InitialCondition=1.04  SampleTime=Ts  HasFrameUpgradeWarning=on
  Unit Delay2 : UnitDelay  InitialCondition=1  SampleTime=Ts  HasFrameUpgradeWarning=on
  Vref : Constant  Value=1.04
  pu : PMIOPort  Side=Left
  fd+ : PMIOPort  Port=2  Side=Right
  fd- : PMIOPort  Port=3  Side=Right
  wires:
  Unit Delay2/1 -> SM PSS1A/1
  PS-Simulink Converter2/1 -> Unit Delay2/1
  Unit Delay1/1 -> SM AC1C/3
  Vref/1 -> SM AC1C/1
  Constant/1 -> SM AC1C/9, SM AC1C/8, SM AC1C/7, SM AC1C/6, SM AC1C/5, SM AC1C/4
  Unit Delay/1 -> SM AC1C/10
  SM AC1C/1 -> Simulink-PS Converter/1
  PS-Simulink Converter1/1 -> Unit Delay/1
  SM PSS1A/1 -> SM AC1C/2
  PS-Simulink Converter/1 -> Unit Delay1/1
  connections:
  PS-Simulink Converter2/LConn1 -- Rotor velocity measurement/RConn1
  Rotor velocity measurement/LConn1 -- Terminal voltage measurement/LConn1 -- pu/RConn1
  Terminal voltage measurement/RConn1 -- PS-Simulink Converter/LConn1
  Synchronous Machine Field Circuit (pu)/LConn1 -- Simulink-PS Converter/RConn1
  Synchronous Machine Field Circuit (pu)/LConn2 -- PS-Simulink Converter1/LConn1
  Synchronous Machine Field Circuit (pu)/RConn2 -- fd-/RConn1
  Synchronous Machine Field Circuit (pu)/RConn1 -- fd+/RConn1

== system pll_stability_9bus/Gen1@Bus1 Swing/Governor and Prime Mover ==
  "Governor and Prime Mover " : Subsystem  mask(Governor and Prime Mover){droop_percentage=5, Tg=0.15, Tch=0.3, pu_torque0=0.309487, Ts=Ts}
      mask prompts: droop_percentage "Percentage droop, (%)"; Tg "Time constant of governor, Tg (s)"; Tch "Time constant of main inlet volumes and steam chest, Tch (s)"; pu_torque0 "Initial torque, (pu)"; Ts "Sample time"
      mask help:
      | Implements a synchronous machine governor and prime mover. The prime mover is a non-reheat steam turbine.
      |
      | The input to the block is a per-unit synchronous machine measurement vector.
      |
      | R and C are mechanical rotational ports.
  Mechanical Power : ee_lib/Electromechanical/Mechanical/Machine Mechanical Power  power_sign=-1  SRated=247.5 MW  FRated=60 Hz  nPolePairs=20  inputUnit=ee.enum.unit.pu  torque_factor=2  inertia_option=2  J=27548 kg*m^2  H=6 W*s/(A*V)  damper_option=2  D=39.0509 N*m*s/rad  pu_D=0  initialization_option=2  fMechanical0=60 Hz  fElectrical0=60 Hz
      settings: InternalSimscapePortConfiguration="{\"Bottom\":[],\"Left\":[{\"id\":\"Pm_pu\",\"label\":\"pu\",\"type\":\"input\"}],\"Right\":[{\"id\":\"R\",\"label\":\"R\",\"type\":\"foundation.mechanical.rotational.rotational\"},{\"id\":\"C\",\"label\":\"C\",\"type\":\"foundation.mechanical.rotational.rotational\"}],\"Top\":[]}"
  PS-Simulink Converter : nesl_utility/PS-Simulink Converter  PhysicalDomain=network_engine_domain  SubClassName=ps_output  LeftPortType=input  RightPortType=output  PseudoPeriodic=off  Frequencies=[]  VectorFormat=1-D array  Unit=1  AffineConversion=off
  Pref : Constant  Value=76.4/247.5
  Rotor velocity measurement : ee_lib/Electromechanical/Synchronous/Synchronous Machine Measurement  output_idx=4
      settings: InternalSimscapePortConfiguration="{\"Bottom\":[],\"Left\":[{\"id\":\"pu_input\",\"label\":\"pu\",\"type\":\"input\"}],\"Right\":[{\"id\":\"pu_output\",\"label\":\"o\",\"type\":\"output\"}],\"Top\":[]}"
  Simulink-PS Converter : nesl_utility/Simulink-PS Converter  PhysicalDomain=network_engine_domain  SubClassName=ps_input  LeftPortType=input  RightPortType=output  PseudoPeriodic=off  Frequencies=[]  NoiseDistribution=none  NoiseParameters=[]  Unit=1  AffineConversion=off  FilteringAndDerivatives=provide  SimscapeFilterOrder=1  InputFilterTimeConstant=0.001  UdotUserProvided=0
  Unit Delay : UnitDelay  InitialCondition=1  SampleTime=Ts  HasFrameUpgradeWarning=on
  wref : Constant
  R : PMIOPort  Side=Right
  C : PMIOPort  Port=2  Side=Right
  pu : PMIOPort  Port=3  Side=Left
  wires:
  PS-Simulink Converter/1 -> Unit Delay/1
  Unit Delay/1 -> "Governor and Prime Mover "/3(w)
  Pref/1 -> "Governor and Prime Mover "/2(Pref)
  "Governor and Prime Mover "/1(Tm) -> Simulink-PS Converter/1
  wref/1 -> "Governor and Prime Mover "/1(wref)
  connections:
  PS-Simulink Converter/LConn1 -- Rotor velocity measurement/RConn1
  Mechanical Power/RConn1 -- R/RConn1
  pu/RConn1 -- Rotor velocity measurement/LConn1
  Mechanical Power/RConn2 -- C/RConn1
  Mechanical Power/LConn1 -- Simulink-PS Converter/RConn1

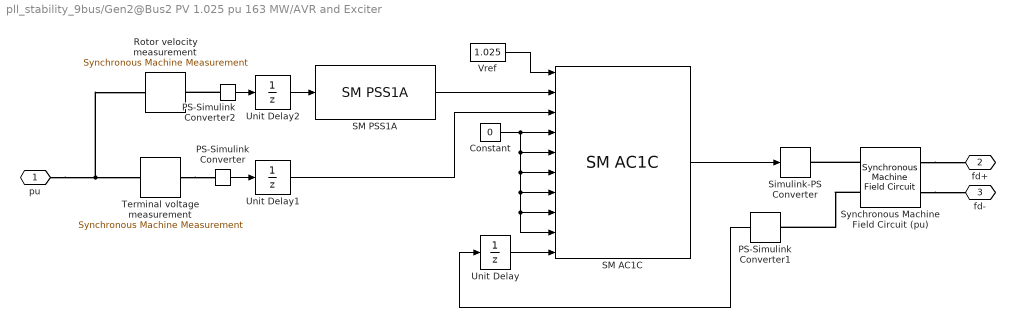
== system pll_stability_9bus/Gen2@Bus2 PV 1.025 pu 163 MW/AVR and Exciter ==
  Constant : Constant  Value=0
  PS-Simulink Converter : nesl_utility/PS-Simulink Converter  PhysicalDomain=network_engine_domain  SubClassName=ps_output  LeftPortType=input  RightPortType=output  PseudoPeriodic=off  Frequencies=[]  VectorFormat=1-D array  Unit=1  AffineConversion=off
  PS-Simulink Converter1 : nesl_utility/PS-Simulink Converter  PhysicalDomain=network_engine_domain  SubClassName=ps_output  LeftPortType=input  RightPortType=output  PseudoPeriodic=off  Frequencies=[]  VectorFormat=1-D array  Unit=1  AffineConversion=off
  PS-Simulink Converter2 : nesl_utility/PS-Simulink Converter  PhysicalDomain=network_engine_domain  SubClassName=ps_output  LeftPortType=input  RightPortType=output  PseudoPeriodic=off  Frequencies=[]  VectorFormat=1-D array  Unit=1  AffineConversion=off
  Rotor velocity measurement : ee_lib/Electromechanical/Synchronous/Synchronous Machine Measurement  output_idx=4
      settings: InternalSimscapePortConfiguration="{\"Bottom\":[],\"Left\":[{\"id\":\"pu_input\",\"label\":\"pu\",\"type\":\"input\"}],\"Right\":[{\"id\":\"pu_output\",\"label\":\"o\",\"type\":\"output\"}],\"Top\":[]}"
  SM AC1C : eeSmAC1C/SM AC1C  E_FD0=1.79759  Ts=Ts  R_C=0  X_C=0  T_R=0  K_A=400  T_A=0.02  T_B=0  T_C=0  K_F=0.03  T_F=1  V_Amax=14.5  V_Amin=-14.5  E_FEmax=6.03  E_FEmin=-5.43  oelInputLocation=Unused  uelInputLocation=Unused  sclInputLocation=Unused  K_E=1  T_E=0.8  K_C=0.2  K_D=0.38  E_1=4.18  S_E_E1=0.1  E_2=3.14  S_E_E2=0.03  V_FEmax=99  V_Emin=0
  SM PSS1A : eeSmPSS1A/SM PSS1A  K_S=3.15  A_1=0  A_2=0  T_1=0  T_2=0  T_3=0.32  T_4=0.016  T_5=1  T_6=0.0106  V_STmax=0.09  V_STmin=-0.09  Ts=Ts
  Simulink-PS Converter : nesl_utility/Simulink-PS Converter  PhysicalDomain=network_engine_domain  SubClassName=ps_input  LeftPortType=input  RightPortType=output  PseudoPeriodic=off  Frequencies=[]  NoiseDistribution=none  NoiseParameters=[]  Unit=1  AffineConversion=off  FilteringAndDerivatives=provide  SimscapeFilterOrder=1  InputFilterTimeConstant=0.001  UdotUserProvided=0
  Synchronous Machine Field Circuit (pu) : ee_lib/Electromechanical/Synchronous/Synchronous Machine Field Circuit  unit_option=ee.enum.unit.pu  SRated=192 MW  FRated=60 Hz  fieldCircuitParameterization_option=ee.enum.sm.fieldparameterization.current  baseEfd=92.95 V  baseIfd=100 A  parameterization_option=ee.enum.sm.parameterization.standard  Ladu=1.6801  Rfd=8.558e-4  Xl=0.1  Xd=1.7199  Xdd=0.23  Xddd=0.1728  d_option=ee.enum.circuit.open  Td0d=6 s  Tdd=1.3260 s  Td0dd=0.05 s  Tddd=0.0230 s
      settings: InternalSimscapePortConfiguration="{\"Bottom\":[],\"Left\":[{\"id\":\"Efd_pu\",\"label\":\"Efd_pu\",\"type\":\"input\"},{\"id\":\"Ifd_pu\",\"label\":\"Ifd_pu\",\"type\":\"output\"}],\"Right\":[{\"id\":\"fd_p\",\"label\":\"fd+\",\"type\":\"foundation.electrical.electrical\"},{\"id\":\"fd_n\",\"label\":\"fd-\",\"type\":\"foundation.electrical.electrical\"}],\"Top\":[]}"
  Terminal voltage measurement : ee_lib/Electromechanical/Synchronous/Synchronous Machine Measurement  output_idx=14
      settings: InternalSimscapePortConfiguration="{\"Bottom\":[],\"Left\":[{\"id\":\"pu_input\",\"label\":\"pu\",\"type\":\"input\"}],\"Right\":[{\"id\":\"pu_output\",\"label\":\"o\",\"type\":\"output\"}],\"Top\":[]}"
  Unit Delay : UnitDelay  InitialCondition=1.79759  SampleTime=Ts  HasFrameUpgradeWarning=on
  Unit Delay1 : UnitDelay  InitialCondition=1.025  SampleTime=Ts  HasFrameUpgradeWarning=on
  Unit Delay2 : UnitDelay  InitialCondition=1  SampleTime=Ts  HasFrameUpgradeWarning=on
  Vref : Constant  Value=1.025
  pu : PMIOPort  Side=Left
  fd+ : PMIOPort  Port=2  Side=Right
  fd- : PMIOPort  Port=3  Side=Right
  wires:
  PS-Simulink Converter/1 -> Unit Delay1/1
  SM PSS1A/1 -> SM AC1C/2
  PS-Simulink Converter1/1 -> Unit Delay/1
  SM AC1C/1 -> Simulink-PS Converter/1
  Unit Delay/1 -> SM AC1C/10
  Constant/1 -> SM AC1C/4, SM AC1C/5, SM AC1C/6, SM AC1C/7, SM AC1C/8, SM AC1C/9
  Vref/1 -> SM AC1C/1
  Unit Delay1/1 -> SM AC1C/3
  Unit Delay2/1 -> SM PSS1A/1
  PS-Simulink Converter2/1 -> Unit Delay2/1
  connections:
  Synchronous Machine Field Circuit (pu)/RConn1 -- fd+/RConn1
  Synchronous Machine Field Circuit (pu)/RConn2 -- fd-/RConn1
  Synchronous Machine Field Circuit (pu)/LConn2 -- PS-Simulink Converter1/LConn1
  Synchronous Machine Field Circuit (pu)/LConn1 -- Simulink-PS Converter/RConn1
  Terminal voltage measurement/RConn1 -- PS-Simulink Converter/LConn1
  pu/RConn1 -- Terminal voltage measurement/LConn1 -- Rotor velocity measurement/LConn1
  PS-Simulink Converter2/LConn1 -- Rotor velocity measurement/RConn1

== system pll_stability_9bus/Gen2@Bus2 PV 1.025 pu 163 MW/Governor and Prime Mover ==
  "Governor and Prime Mover " : Subsystem  mask(Governor and Prime Mover){droop_percentage=5, Tg=0.15, Tch=0.3, pu_torque0=0.855832, Ts=Ts}
      mask prompts: droop_percentage "Percentage droop, (%)"; Tg "Time constant of governor, Tg (s)"; Tch "Time constant of main inlet volumes and steam chest, Tch (s)"; pu_torque0 "Initial torque, (pu)"; Ts "Sample time"
      mask help:
      | Implements a synchronous machine governor and prime mover. The prime mover is a non-reheat steam turbine.
      |
      | The input to the block is a per-unit synchronous machine measurement vector.
      |
      | R and C are mechanical rotational ports.
  Mechanical Power : ee_lib/Electromechanical/Mechanical/Machine Mechanical Power  power_sign=-1  SRated=192 MW  FRated=60 Hz  nPolePairs=1  inputUnit=ee.enum.unit.pu  torque_factor=2  inertia_option=2  J=27548 kg*m^2  H=3.3333 W*s/(A*V)  damper_option=2  D=39.0509 N*m*s/rad  pu_D=0  initialization_option=2  fMechanical0=60 Hz  fElectrical0=60 Hz
      settings: InternalSimscapePortConfiguration="{\"Bottom\":[],\"Left\":[{\"id\":\"Pm_pu\",\"label\":\"pu\",\"type\":\"input\"}],\"Right\":[{\"id\":\"R\",\"label\":\"R\",\"type\":\"foundation.mechanical.rotational.rotational\"},{\"id\":\"C\",\"label\":\"C\",\"type\":\"foundation.mechanical.rotational.rotational\"}],\"Top\":[]}"
  PS-Simulink Converter : nesl_utility/PS-Simulink Converter  PhysicalDomain=network_engine_domain  SubClassName=ps_output  LeftPortType=input  RightPortType=output  PseudoPeriodic=off  Frequencies=[]  VectorFormat=1-D array  Unit=1  AffineConversion=off
  Pref : Constant  Value=163/192
  Rotor velocity measurement : ee_lib/Electromechanical/Synchronous/Synchronous Machine Measurement  output_idx=4
      settings: InternalSimscapePortConfiguration="{\"Bottom\":[],\"Left\":[{\"id\":\"pu_input\",\"label\":\"pu\",\"type\":\"input\"}],\"Right\":[{\"id\":\"pu_output\",\"label\":\"o\",\"type\":\"output\"}],\"Top\":[]}"
  Simulink-PS Converter : nesl_utility/Simulink-PS Converter  PhysicalDomain=network_engine_domain  SubClassName=ps_input  LeftPortType=input  RightPortType=output  PseudoPeriodic=off  Frequencies=[]  NoiseDistribution=none  NoiseParameters=[]  Unit=1  AffineConversion=off  FilteringAndDerivatives=provide  SimscapeFilterOrder=1  InputFilterTimeConstant=0.001  UdotUserProvided=0
  Unit Delay : UnitDelay  InitialCondition=1  SampleTime=Ts  HasFrameUpgradeWarning=on
  wref : Constant
  R : PMIOPort  Side=Right
  C : PMIOPort  Port=2  Side=Right
  pu : PMIOPort  Port=3  Side=Left
  wires:
  wref/1 -> "Governor and Prime Mover "/1(wref)
  "Governor and Prime Mover "/1(Tm) -> Simulink-PS Converter/1
  Pref/1 -> "Governor and Prime Mover "/2(Pref)
  Unit Delay/1 -> "Governor and Prime Mover "/3(w)
  PS-Simulink Converter/1 -> Unit Delay/1
  connections:
  Mechanical Power/LConn1 -- Simulink-PS Converter/RConn1
  Mechanical Power/RConn2 -- C/RConn1
  pu/RConn1 -- Rotor velocity measurement/LConn1
  Mechanical Power/RConn1 -- R/RConn1
  PS-Simulink Converter/LConn1 -- Rotor velocity measurement/RConn1

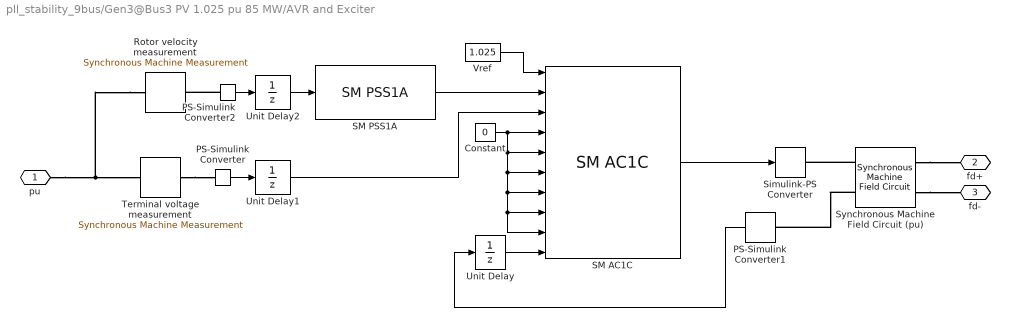
== system pll_stability_9bus/Gen3@Bus3 PV 1.025 pu 85 MW/AVR and Exciter ==
  Constant : Constant  Value=0
  PS-Simulink Converter : nesl_utility/PS-Simulink Converter  PhysicalDomain=network_engine_domain  SubClassName=ps_output  LeftPortType=input  RightPortType=output  PseudoPeriodic=off  Frequencies=[]  VectorFormat=1-D array  Unit=1  AffineConversion=off
  PS-Simulink Converter1 : nesl_utility/PS-Simulink Converter  PhysicalDomain=network_engine_domain  SubClassName=ps_output  LeftPortType=input  RightPortType=output  PseudoPeriodic=off  Frequencies=[]  VectorFormat=1-D array  Unit=1  AffineConversion=off
  PS-Simulink Converter2 : nesl_utility/PS-Simulink Converter  PhysicalDomain=network_engine_domain  SubClassName=ps_output  LeftPortType=input  RightPortType=output  PseudoPeriodic=off  Frequencies=[]  VectorFormat=1-D array  Unit=1  AffineConversion=off
  Rotor velocity measurement : ee_lib/Electromechanical/Synchronous/Synchronous Machine Measurement  output_idx=4
      settings: InternalSimscapePortConfiguration="{\"Bottom\":[],\"Left\":[{\"id\":\"pu_input\",\"label\":\"pu\",\"type\":\"input\"}],\"Right\":[{\"id\":\"pu_output\",\"label\":\"o\",\"type\":\"output\"}],\"Top\":[]}"
  SM AC1C : eeSmAC1C/SM AC1C  E_FD0=1.41658  Ts=Ts  R_C=0  X_C=0  T_R=0  K_A=400  T_A=0.02  T_B=0  T_C=0  K_F=0.03  T_F=1  V_Amax=14.5  V_Amin=-14.5  E_FEmax=6.03  E_FEmin=-5.43  oelInputLocation=Unused  uelInputLocation=Unused  sclInputLocation=Unused  K_E=1  T_E=0.8  K_C=0.2  K_D=0.38  E_1=4.18  S_E_E1=0.1  E_2=3.14  S_E_E2=0.03  V_FEmax=99  V_Emin=0
  SM PSS1A : eeSmPSS1A/SM PSS1A  K_S=3.15  A_1=0  A_2=0  T_1=0  T_2=0  T_3=0.32  T_4=0.016  T_5=1  T_6=0.0106  V_STmax=0.09  V_STmin=-0.09  Ts=Ts
  Simulink-PS Converter : nesl_utility/Simulink-PS Converter  PhysicalDomain=network_engine_domain  SubClassName=ps_input  LeftPortType=input  RightPortType=output  PseudoPeriodic=off  Frequencies=[]  NoiseDistribution=none  NoiseParameters=[]  Unit=1  AffineConversion=off  FilteringAndDerivatives=provide  SimscapeFilterOrder=1  InputFilterTimeConstant=0.001  UdotUserProvided=0
  Synchronous Machine Field Circuit (pu) : ee_lib/Electromechanical/Synchronous/Synchronous Machine Field Circuit  unit_option=ee.enum.unit.pu  SRated=128 MW  FRated=60 Hz  fieldCircuitParameterization_option=ee.enum.sm.fieldparameterization.current  baseEfd=92.95 V  baseIfd=100 A  parameterization_option=ee.enum.sm.parameterization.standard  Ladu=1.5958  Rfd=8.4749e-4  Xl=0.095  Xd=1.68  Xdd=0.2321  Xddd=0.128  d_option=ee.enum.circuit.open  Td0d=5.89 s  Tdd=1.3260 s  Td0dd=0.05 s  Tddd=0.0230 s
      settings: InternalSimscapePortConfiguration="{\"Bottom\":[],\"Left\":[{\"id\":\"Efd_pu\",\"label\":\"Efd_pu\",\"type\":\"input\"},{\"id\":\"Ifd_pu\",\"label\":\"Ifd_pu\",\"type\":\"output\"}],\"Right\":[{\"id\":\"fd_p\",\"label\":\"fd+\",\"type\":\"foundation.electrical.electrical\"},{\"id\":\"fd_n\",\"label\":\"fd-\",\"type\":\"foundation.electrical.electrical\"}],\"Top\":[]}"
  Terminal voltage measurement : ee_lib/Electromechanical/Synchronous/Synchronous Machine Measurement  output_idx=14
      settings: InternalSimscapePortConfiguration="{\"Bottom\":[],\"Left\":[{\"id\":\"pu_input\",\"label\":\"pu\",\"type\":\"input\"}],\"Right\":[{\"id\":\"pu_output\",\"label\":\"o\",\"type\":\"output\"}],\"Top\":[]}"
  Unit Delay : UnitDelay  InitialCondition=1.41658  SampleTime=Ts  HasFrameUpgradeWarning=on
  Unit Delay1 : UnitDelay  InitialCondition=1.025  SampleTime=Ts  HasFrameUpgradeWarning=on
  Unit Delay2 : UnitDelay  InitialCondition=1  SampleTime=Ts  HasFrameUpgradeWarning=on
  Vref : Constant  Value=1.025
  pu : PMIOPort  Side=Left
  fd+ : PMIOPort  Port=2  Side=Right
  fd- : PMIOPort  Port=3  Side=Right
  wires:
  Unit Delay2/1 -> SM PSS1A/1
  PS-Simulink Converter2/1 -> Unit Delay2/1
  Unit Delay1/1 -> SM AC1C/3
  Vref/1 -> SM AC1C/1
  Constant/1 -> SM AC1C/9, SM AC1C/8, SM AC1C/7, SM AC1C/6, SM AC1C/5, SM AC1C/4
  Unit Delay/1 -> SM AC1C/10
  SM AC1C/1 -> Simulink-PS Converter/1
  PS-Simulink Converter1/1 -> Unit Delay/1
  SM PSS1A/1 -> SM AC1C/2
  PS-Simulink Converter/1 -> Unit Delay1/1
  connections:
  PS-Simulink Converter2/LConn1 -- Rotor velocity measurement/RConn1
  Rotor velocity measurement/LConn1 -- Terminal voltage measurement/LConn1 -- pu/RConn1
  Terminal voltage measurement/RConn1 -- PS-Simulink Converter/LConn1
  Synchronous Machine Field Circuit (pu)/LConn1 -- Simulink-PS Converter/RConn1
  Synchronous Machine Field Circuit (pu)/LConn2 -- PS-Simulink Converter1/LConn1
  Synchronous Machine Field Circuit (pu)/RConn2 -- fd-/RConn1
  Synchronous Machine Field Circuit (pu)/RConn1 -- fd+/RConn1
